simulink model "pattern_separation"  (R2019b)
settings: Solver=FixedStepAuto  StartTime=1  StopTime=simulationtime  FixedStep=stepsize  RelTol=1e-3
values from neighbouring files (symbols this model uses):
  a1 = 0.02    [simulation.m]
  a2 = 0.02    [simulation.m]
  b1 = 0.025    [simulation.m]
  b2 = 0.04    [simulation.m]
  c1 = -65    [simulation.m]
  C1 = normrnd(100,10,[1,nrofgranulecells])    [simulation.m]
  c2 = -65    [simulation.m]
  C2 = normrnd(100,10,[1,nrofinterneurons])    [simulation.m]
  d1 = 6    [simulation.m]
  d2 = 2    [simulation.m]
  inputset = inputsets{no_input}    [simulation.m]
  k1 = 0.25    [simulation.m]
  k2 = 0.25    [simulation.m]
  minimum_saturation_limit_1 = -80    [simulation.m]
  minimum_saturation_limit_2 = -100    [simulation.m]
  noumberofevents = 500    [simulation.m]
  Re = 230    [simulation.m]
  simulationtime = 2000    [simulation.m]
  stepsize = 1    [simulation.m]
  ve1 = -5    [simulation.m]
  ve2 = -80    [simulation.m]
  vr1 = -60    [simulation.m]
  vr2 = -65    [simulation.m]
  vt1 = -55    [simulation.m]
  vt2 = -48    [simulation.m]
undefined symbols (not defined in the file or in its folder): conductancemaxima1, conductancemaxima2, conductancemaxima3, decaytimes1, decaytimes2, decaytimes3, DiscIntNeverNeededParam, Nd, trace
(part 4 of 5)

== system pattern_separation/granule cell 20/GC neuron ==
  postsynaptic current : Inport
  AHP or ADP : Constant  Value=c1  SampleTime=-1
  AP threshold potential : Constant  Value=vt1  SampleTime=-1
  Add : Sum  Inputs=+-
  Add2 : Sum  Inputs=+-
  Add3 : Sum  Inputs=+-
  Constant1 : Constant  Value=d1  SampleTime=-1
  Gain1 : Gain  Gain=b1
  Gain2 : Gain  Gain=k1
  Integrator : Integrator  ExternalReset=rising  InitialCondition=d1
  Integrator1 : Integrator  ExternalReset=rising  InitialCondition=vr1  LimitOutput=on  UpperSaturationLimit=30  LowerSaturationLimit=minimum_saturation_limit_1
  Memory : Memory  InheritSampleTime=on
  Memory1 : Memory  InitialCondition=vr1  InheritSampleTime=on
  Product : Product
  f' : Sum  Inputs=++-
  f'' : Sum  Inputs=+-
  membrne capacitance : Gain  Gain=1/C1(20)
  reset function : MATLAB Function  TreatAsAtomicUnit=on
  resting membrane potential : Constant  Value=vr1  SampleTime=-1
  time constant of relative refractory period : Gain  Gain=a1
  v : Outport
  output : Outport  Port=2
  wires:
  time constant of relative refractory period/1 -> Integrator/1  "u"
  Constant1/1 -> reset function/3(d)
  f''/1 -> time constant of relative refractory period/1
  membrne capacitance/1 -> Integrator1/1  "v"
  resting membrane potential/1 -> Add2/2, Add/2
  AHP or ADP/1 -> reset function/2(c)
  Add2/1 -> Product/1
  reset function/3(r) -> Integrator1/2, Integrator/2, output/1
  Gain1/1 -> f''/1
  Add3/1 -> Product/2
  Memory1/1 -> reset function/1(v)
  reset function/1(v1) -> Add/1, Add2/1, Add3/1
  reset function/2(u1) -> f''/2, f'/3
  Memory/1 -> reset function/4(u)
  Add/1 -> Gain1/1
  Integrator/1 -> Memory/1  "u"
  AP threshold potential/1 -> Add3/2
  Integrator1/1 -> v/1, Memory1/1  "v"
  f'/1 -> membrne capacitance/1
  Product/1 -> Gain2/1
  Gain2/1 -> f'/2
  postsynaptic current/1 -> f'/1

== system pattern_separation/granule cell 20/single exp EPSCs generator (recurrent synapse) ==
  event time : Inport
  decay time constant : Inport  Port=2
  conductance maximum : Inport  Port=3
  Add1 : Sum  Inputs=+-
  MATLAB Function : MATLAB Function  TreatAsAtomicUnit=on
  Multiply : Gain  Gain=-1
  Product : Product
  Product1 : Product  Inputs=*/
  Product2 : Product
  current reversal potential : Constant  Value=ve1  SampleTime=-1
  resting membrane potential : Constant  Value=vr1  SampleTime=-1
  postsynaptic current : Outport
  wires:
  decay time constant/1 -> Product1/2
  Product/1 -> postsynaptic current/1  "postsynaptic current"
  resting membrane potential/1 -> Add1/1
  current reversal potential/1 -> Add1/2
  conductance maximum/1 -> Product2/2
  Product2/1 -> Product/2  "conductance"
  Add1/1 -> Multiply/1
  Product1/1 -> MATLAB Function/1(inp)
  MATLAB Function/1(exponential) -> Product2/1
  event time/1 -> Product1/1
  Multiply/1 -> Product/1

== system pattern_separation/granule cell 20/single exp IPSCs generator (ihibitory synapse) ==
  event time : Inport
  decay time constant : Inport  Port=2
  conductance maximum : Inport  Port=3
  Add1 : Sum  Inputs=+-
  MATLAB Function : MATLAB Function  TreatAsAtomicUnit=on
  Multiply : Gain  Gain=-1
  Product : Product
  Product1 : Product  Inputs=*/
  Product2 : Product
  current reversal potential : Constant  Value=ve2  SampleTime=-1
  resting membrane potential : Constant  Value=vr2  SampleTime=-1
  postsynaptic current : Outport
  wires:
  decay time constant/1 -> Product1/2
  Product/1 -> postsynaptic current/1  "postsynaptic current"
  resting membrane potential/1 -> Add1/1
  current reversal potential/1 -> Add1/2
  conductance maximum/1 -> Product2/2
  Product2/1 -> Product/2  "conductance"
  Add1/1 -> Multiply/1
  Product1/1 -> MATLAB Function/1(inp)
  MATLAB Function/1(exponential) -> Product2/1
  event time/1 -> Product1/1
  Multiply/1 -> Product/1

== system pattern_separation/granule cell 3/GC neuron ==
  postsynaptic current : Inport
  AHP or ADP : Constant  Value=c1  SampleTime=-1
  AP threshold potential : Constant  Value=vt1  SampleTime=-1
  Add : Sum  Inputs=+-
  Add2 : Sum  Inputs=+-
  Add3 : Sum  Inputs=+-
  Constant1 : Constant  Value=d1  SampleTime=-1
  Gain1 : Gain  Gain=b1
  Gain2 : Gain  Gain=k1
  Integrator : Integrator  ExternalReset=rising  InitialCondition=d1
  Integrator1 : Integrator  ExternalReset=rising  InitialCondition=vr1  LimitOutput=on  UpperSaturationLimit=30  LowerSaturationLimit=minimum_saturation_limit_1
  Memory : Memory  InheritSampleTime=on
  Memory1 : Memory  InitialCondition=vr1  InheritSampleTime=on
  Product : Product
  f' : Sum  Inputs=++-
  f'' : Sum  Inputs=+-
  membrne capacitance : Gain  Gain=1/C1(3)
  reset function : MATLAB Function  TreatAsAtomicUnit=on
  resting membrane potential : Constant  Value=vr1  SampleTime=-1
  time constant of relative refractory period : Gain  Gain=a1
  v : Outport
  output : Outport  Port=2
  wires:
  time constant of relative refractory period/1 -> Integrator/1  "u"
  Constant1/1 -> reset function/3(d)
  f''/1 -> time constant of relative refractory period/1
  membrne capacitance/1 -> Integrator1/1  "v"
  resting membrane potential/1 -> Add2/2, Add/2
  AHP or ADP/1 -> reset function/2(c)
  Add2/1 -> Product/1
  reset function/3(r) -> Integrator1/2, Integrator/2, output/1
  Gain1/1 -> f''/1
  Add3/1 -> Product/2
  Memory1/1 -> reset function/1(v)
  reset function/1(v1) -> Add/1, Add2/1, Add3/1
  reset function/2(u1) -> f''/2, f'/3
  Memory/1 -> reset function/4(u)
  Add/1 -> Gain1/1
  Integrator/1 -> Memory/1  "u"
  AP threshold potential/1 -> Add3/2
  Integrator1/1 -> v/1, Memory1/1  "v"
  f'/1 -> membrne capacitance/1
  Product/1 -> Gain2/1
  Gain2/1 -> f'/2
  postsynaptic current/1 -> f'/1

== system pattern_separation/granule cell 3/single exp EPSCs generator (recurrent synapse) ==
  event time : Inport
  decay time constant : Inport  Port=2
  conductance maximum : Inport  Port=3
  Add1 : Sum  Inputs=+-
  MATLAB Function : MATLAB Function  TreatAsAtomicUnit=on
  Multiply : Gain  Gain=-1
  Product : Product
  Product1 : Product  Inputs=*/
  Product2 : Product
  current reversal potential : Constant  Value=ve1  SampleTime=-1
  resting membrane potential : Constant  Value=vr1  SampleTime=-1
  postsynaptic current : Outport
  wires:
  decay time constant/1 -> Product1/2
  Product/1 -> postsynaptic current/1  "postsynaptic current"
  resting membrane potential/1 -> Add1/1
  current reversal potential/1 -> Add1/2
  conductance maximum/1 -> Product2/2
  Product2/1 -> Product/2  "conductance"
  Add1/1 -> Multiply/1
  Product1/1 -> MATLAB Function/1(inp)
  MATLAB Function/1(exponential) -> Product2/1
  event time/1 -> Product1/1
  Multiply/1 -> Product/1

== system pattern_separation/granule cell 3/single exp IPSCs generator (ihibitory synapse) ==
  event time : Inport
  decay time constant : Inport  Port=2
  conductance maximum : Inport  Port=3
  Add1 : Sum  Inputs=+-
  MATLAB Function : MATLAB Function  TreatAsAtomicUnit=on
  Multiply : Gain  Gain=-1
  Product : Product
  Product1 : Product  Inputs=*/
  Product2 : Product
  current reversal potential : Constant  Value=ve2  SampleTime=-1
  resting membrane potential : Constant  Value=vr2  SampleTime=-1
  postsynaptic current : Outport
  wires:
  decay time constant/1 -> Product1/2
  Product/1 -> postsynaptic current/1  "postsynaptic current"
  resting membrane potential/1 -> Add1/1
  current reversal potential/1 -> Add1/2
  conductance maximum/1 -> Product2/2
  Product2/1 -> Product/2  "conductance"
  Add1/1 -> Multiply/1
  Product1/1 -> MATLAB Function/1(inp)
  MATLAB Function/1(exponential) -> Product2/1
  event time/1 -> Product1/1
  Multiply/1 -> Product/1

== system pattern_separation/granule cell 4/GC neuron ==
  postsynaptic current : Inport
  AHP or ADP : Constant  Value=c1  SampleTime=-1
  AP threshold potential : Constant  Value=vt1  SampleTime=-1
  Add : Sum  Inputs=+-
  Add2 : Sum  Inputs=+-
  Add3 : Sum  Inputs=+-
  Constant1 : Constant  Value=d1  SampleTime=-1
  Gain1 : Gain  Gain=b1
  Gain2 : Gain  Gain=k1
  Integrator : Integrator  ExternalReset=rising  InitialCondition=d1
  Integrator1 : Integrator  ExternalReset=rising  InitialCondition=vr1  LimitOutput=on  UpperSaturationLimit=30  LowerSaturationLimit=minimum_saturation_limit_1
  Memory : Memory  InheritSampleTime=on
  Memory1 : Memory  InitialCondition=vr1  InheritSampleTime=on
  Product : Product
  f' : Sum  Inputs=++-
  f'' : Sum  Inputs=+-
  membrne capacitance : Gain  Gain=1/C1(4)
  reset function : MATLAB Function  TreatAsAtomicUnit=on
  resting membrane potential : Constant  Value=vr1  SampleTime=-1
  time constant of relative refractory period : Gain  Gain=a1
  v : Outport
  output : Outport  Port=2
  wires:
  time constant of relative refractory period/1 -> Integrator/1  "u"
  Constant1/1 -> reset function/3(d)
  f''/1 -> time constant of relative refractory period/1
  membrne capacitance/1 -> Integrator1/1  "v"
  resting membrane potential/1 -> Add2/2, Add/2
  AHP or ADP/1 -> reset function/2(c)
  Add2/1 -> Product/1
  reset function/3(r) -> Integrator1/2, Integrator/2, output/1
  Gain1/1 -> f''/1
  Add3/1 -> Product/2
  Memory1/1 -> reset function/1(v)
  reset function/1(v1) -> Add/1, Add2/1, Add3/1
  reset function/2(u1) -> f''/2, f'/3
  Memory/1 -> reset function/4(u)
  Add/1 -> Gain1/1
  Integrator/1 -> Memory/1  "u"
  AP threshold potential/1 -> Add3/2
  Integrator1/1 -> v/1, Memory1/1  "v"
  f'/1 -> membrne capacitance/1
  Product/1 -> Gain2/1
  Gain2/1 -> f'/2
  postsynaptic current/1 -> f'/1

== system pattern_separation/granule cell 4/single exp EPSCs generator (recurrent synapse) ==
  event time : Inport
  decay time constant : Inport  Port=2
  conductance maximum : Inport  Port=3
  Add1 : Sum  Inputs=+-
  MATLAB Function : MATLAB Function  TreatAsAtomicUnit=on
  Multiply : Gain  Gain=-1
  Product : Product
  Product1 : Product  Inputs=*/
  Product2 : Product
  current reversal potential : Constant  Value=ve1  SampleTime=-1
  resting membrane potential : Constant  Value=vr1  SampleTime=-1
  postsynaptic current : Outport
  wires:
  decay time constant/1 -> Product1/2
  Product/1 -> postsynaptic current/1  "postsynaptic current"
  resting membrane potential/1 -> Add1/1
  current reversal potential/1 -> Add1/2
  conductance maximum/1 -> Product2/2
  Product2/1 -> Product/2  "conductance"
  Add1/1 -> Multiply/1
  Product1/1 -> MATLAB Function/1(inp)
  MATLAB Function/1(exponential) -> Product2/1
  event time/1 -> Product1/1
  Multiply/1 -> Product/1

== system pattern_separation/granule cell 4/single exp IPSCs generator (ihibitory synapse) ==
  event time : Inport
  decay time constant : Inport  Port=2
  conductance maximum : Inport  Port=3
  Add1 : Sum  Inputs=+-
  MATLAB Function : MATLAB Function  TreatAsAtomicUnit=on
  Multiply : Gain  Gain=-1
  Product : Product
  Product1 : Product  Inputs=*/
  Product2 : Product
  current reversal potential : Constant  Value=ve2  SampleTime=-1
  resting membrane potential : Constant  Value=vr2  SampleTime=-1
  postsynaptic current : Outport
  wires:
  decay time constant/1 -> Product1/2
  Product/1 -> postsynaptic current/1  "postsynaptic current"
  resting membrane potential/1 -> Add1/1
  current reversal potential/1 -> Add1/2
  conductance maximum/1 -> Product2/2
  Product2/1 -> Product/2  "conductance"
  Add1/1 -> Multiply/1
  Product1/1 -> MATLAB Function/1(inp)
  MATLAB Function/1(exponential) -> Product2/1
  event time/1 -> Product1/1
  Multiply/1 -> Product/1

== system pattern_separation/granule cell 5/granule cell ==
  postsynaptic current : Inport
  AHP or ADP : Constant  Value=c1  SampleTime=-1
  AP threshold potential : Constant  Value=vt1  SampleTime=-1
  Add : Sum  Inputs=+-
  Add2 : Sum  Inputs=+-
  Add3 : Sum  Inputs=+-
  Constant1 : Constant  Value=d1  SampleTime=-1
  Gain1 : Gain  Gain=b1
  Gain2 : Gain  Gain=k1
  Integrator : Integrator  ExternalReset=rising  InitialCondition=d1
  Integrator1 : Integrator  ExternalReset=rising  InitialCondition=vr1  LimitOutput=on  UpperSaturationLimit=30  LowerSaturationLimit=minimum_saturation_limit_1
  Memory : Memory  InheritSampleTime=on
  Memory1 : Memory  InitialCondition=vr1  InheritSampleTime=on
  Product : Product
  f' : Sum  Inputs=++-
  f'' : Sum  Inputs=+-
  membrne capacitance : Gain  Gain=1/C1(5)
  reset function : MATLAB Function  TreatAsAtomicUnit=on
  resting membrane potential : Constant  Value=vr1  SampleTime=-1
  time constant of relative refractory period : Gain  Gain=a1
  v : Outport
  output : Outport  Port=2
  wires:
  time constant of relative refractory period/1 -> Integrator/1  "u"
  Constant1/1 -> reset function/3(d)
  f''/1 -> time constant of relative refractory period/1
  membrne capacitance/1 -> Integrator1/1  "v"
  resting membrane potential/1 -> Add2/2, Add/2
  AHP or ADP/1 -> reset function/2(c)
  Add2/1 -> Product/1
  reset function/3(r) -> output/1, Integrator1/2, Integrator/2
  Gain1/1 -> f''/1
  Add3/1 -> Product/2
  Memory1/1 -> reset function/1(v)
  reset function/1(v1) -> Add/1, Add2/1, Add3/1
  reset function/2(u1) -> f''/2, f'/3
  Memory/1 -> reset function/4(u)
  Add/1 -> Gain1/1
  Integrator/1 -> Memory/1  "u"
  AP threshold potential/1 -> Add3/2
  Integrator1/1 -> v/1, Memory1/1  "v"
  f'/1 -> membrne capacitance/1
  Product/1 -> Gain2/1
  Gain2/1 -> f'/2
  postsynaptic current/1 -> f'/1

== system pattern_separation/granule cell 5/single exp EPSCs generator (recurrent synapse) ==
  event time : Inport
  decay time constant : Inport  Port=2
  conductance maximum : Inport  Port=3
  Add1 : Sum  Inputs=+-
  MATLAB Function : MATLAB Function  TreatAsAtomicUnit=on
  Multiply : Gain  Gain=-1
  Product : Product
  Product1 : Product  Inputs=*/
  Product2 : Product
  current reversal potential : Constant  Value=ve1  SampleTime=-1
  resting membrane potential : Constant  Value=vr1  SampleTime=-1
  postsynaptic current : Outport
  wires:
  decay time constant/1 -> Product1/2
  Product/1 -> postsynaptic current/1  "postsynaptic current"
  resting membrane potential/1 -> Add1/1
  current reversal potential/1 -> Add1/2
  conductance maximum/1 -> Product2/2
  Product2/1 -> Product/2  "conductance"
  Add1/1 -> Multiply/1
  Product1/1 -> MATLAB Function/1(inp)
  MATLAB Function/1(exponential) -> Product2/1
  event time/1 -> Product1/1
  Multiply/1 -> Product/1

== system pattern_separation/granule cell 5/single exp IPSCs generator (ihibitory synapse) ==
  event time : Inport
  decay time constant : Inport  Port=2
  conductance maximum : Inport  Port=3
  Add1 : Sum  Inputs=+-
  MATLAB Function : MATLAB Function  TreatAsAtomicUnit=on
  Multiply : Gain  Gain=-1
  Product : Product
  Product1 : Product  Inputs=*/
  Product2 : Product
  current reversal potential : Constant  Value=ve2  SampleTime=-1
  resting membrane potential : Constant  Value=vr2  SampleTime=-1
  postsynaptic current : Outport
  wires:
  decay time constant/1 -> Product1/2
  Product/1 -> postsynaptic current/1  "postsynaptic current"
  resting membrane potential/1 -> Add1/1
  current reversal potential/1 -> Add1/2
  conductance maximum/1 -> Product2/2
  Product2/1 -> Product/2  "conductance"
  Add1/1 -> Multiply/1
  Product1/1 -> MATLAB Function/1(inp)
  MATLAB Function/1(exponential) -> Product2/1
  event time/1 -> Product1/1
  Multiply/1 -> Product/1

== system pattern_separation/granule cell 6/GC neuron ==
  postsynaptic current : Inport
  AHP or ADP : Constant  Value=c1  SampleTime=-1
  AP threshold potential : Constant  Value=vt1  SampleTime=-1
  Add : Sum  Inputs=+-
  Add2 : Sum  Inputs=+-
  Add3 : Sum  Inputs=+-
  Constant1 : Constant  Value=d1  SampleTime=-1
  Gain1 : Gain  Gain=b1
  Gain2 : Gain  Gain=k1
  Integrator : Integrator  ExternalReset=rising  InitialCondition=d1
  Integrator1 : Integrator  ExternalReset=rising  InitialCondition=vr1  LimitOutput=on  UpperSaturationLimit=30  LowerSaturationLimit=minimum_saturation_limit_1
  Memory : Memory  InheritSampleTime=on
  Memory1 : Memory  InitialCondition=vr1  InheritSampleTime=on
  Product : Product  RndMeth=Nearest
  f' : Sum  Inputs=++-
  f'' : Sum  Inputs=+-
  membrne capacitance : Gain  Gain=1/C1(6)
  reset function : MATLAB Function  TreatAsAtomicUnit=on
  resting membrane potential : Constant  Value=vr1  SampleTime=-1
  time constant of relative refractory period : Gain  Gain=a1
  v : Outport
  output : Outport  Port=2
  wires:
  time constant of relative refractory period/1 -> Integrator/1  "u"
  Constant1/1 -> reset function/3(d)
  f''/1 -> time constant of relative refractory period/1
  membrne capacitance/1 -> Integrator1/1  "v"
  resting membrane potential/1 -> Add2/2, Add/2
  AHP or ADP/1 -> reset function/2(c)
  Add2/1 -> Product/1
  reset function/3(r) -> Integrator1/2, Integrator/2, output/1
  Gain1/1 -> f''/1
  Add3/1 -> Product/2
  Memory1/1 -> reset function/1(v)
  reset function/1(v1) -> Add/1, Add2/1, Add3/1
  reset function/2(u1) -> f''/2, f'/3
  Memory/1 -> reset function/4(u)
  Add/1 -> Gain1/1
  Integrator/1 -> Memory/1  "u"
  AP threshold potential/1 -> Add3/2
  Integrator1/1 -> v/1, Memory1/1  "v"
  f'/1 -> membrne capacitance/1
  Product/1 -> Gain2/1
  Gain2/1 -> f'/2
  postsynaptic current/1 -> f'/1

== system pattern_separation/granule cell 6/single exp EPSCs generator (recurrent synapse) ==
  event time : Inport
  decay time constant : Inport  Port=2
  conductance maximum : Inport  Port=3
  Add1 : Sum  Inputs=+-
  MATLAB Function : MATLAB Function  TreatAsAtomicUnit=on
  Multiply : Gain  Gain=-1
  Product : Product
  Product1 : Product  Inputs=*/
  Product2 : Product
  current reversal potential : Constant  Value=ve1  SampleTime=-1
  resting membrane potential : Constant  Value=vr1  SampleTime=-1
  postsynaptic current : Outport
  wires:
  decay time constant/1 -> Product1/2
  Product/1 -> postsynaptic current/1  "postsynaptic current"
  resting membrane potential/1 -> Add1/1
  current reversal potential/1 -> Add1/2
  conductance maximum/1 -> Product2/2
  Product2/1 -> Product/2  "conductance"
  Add1/1 -> Multiply/1
  Product1/1 -> MATLAB Function/1(inp)
  MATLAB Function/1(exponential) -> Product2/1
  event time/1 -> Product1/1
  Multiply/1 -> Product/1

== system pattern_separation/granule cell 6/single exp IPSCs generator (ihibitory synapse) ==
  event time : Inport
  decay time constant : Inport  Port=2
  conductance maximum : Inport  Port=3
  Add1 : Sum  Inputs=+-
  MATLAB Function : MATLAB Function  TreatAsAtomicUnit=on
  Multiply : Gain  Gain=-1
  Product : Product
  Product1 : Product  Inputs=*/
  Product2 : Product
  current reversal potential : Constant  Value=ve2  SampleTime=-1
  resting membrane potential : Constant  Value=vr2  SampleTime=-1
  postsynaptic current : Outport
  wires:
  decay time constant/1 -> Product1/2
  Product/1 -> postsynaptic current/1  "postsynaptic current"
  resting membrane potential/1 -> Add1/1
  current reversal potential/1 -> Add1/2
  conductance maximum/1 -> Product2/2
  Product2/1 -> Product/2  "conductance"
  Add1/1 -> Multiply/1
  Product1/1 -> MATLAB Function/1(inp)
  MATLAB Function/1(exponential) -> Product2/1
  event time/1 -> Product1/1
  Multiply/1 -> Product/1

== system pattern_separation/granule cell 7/granule cell ==
  postsynaptic current : Inport
  AHP or ADP : Constant  Value=c1  SampleTime=-1
  AP threshold potential : Constant  Value=vt1  SampleTime=-1
  Add : Sum  Inputs=+-
  Add2 : Sum  Inputs=+-
  Add3 : Sum  Inputs=+-
  Constant1 : Constant  Value=d1  SampleTime=-1
  Gain1 : Gain  Gain=b1
  Gain2 : Gain  Gain=k1
  Integrator : Integrator  ExternalReset=rising  InitialCondition=d1
  Integrator1 : Integrator  ExternalReset=rising  InitialCondition=vr1  LimitOutput=on  UpperSaturationLimit=30  LowerSaturationLimit=minimum_saturation_limit_1
  Memory : Memory  InheritSampleTime=on
  Memory1 : Memory  InitialCondition=vr1  InheritSampleTime=on
  Product : Product
  f' : Sum  Inputs=++-
  f'' : Sum  Inputs=+-
  membrne capacitance : Gain  Gain=1/C1(7)
  reset function : MATLAB Function  TreatAsAtomicUnit=on
  resting membrane potential : Constant  Value=vr1  SampleTime=-1
  time constant of relative refractory period : Gain  Gain=a1
  v : Outport
  output : Outport  Port=2
  wires:
  time constant of relative refractory period/1 -> Integrator/1  "u"
  Constant1/1 -> reset function/3(d)
  f''/1 -> time constant of relative refractory period/1
  membrne capacitance/1 -> Integrator1/1  "v"
  resting membrane potential/1 -> Add2/2, Add/2
  AHP or ADP/1 -> reset function/2(c)
  Add2/1 -> Product/1
  reset function/3(r) -> output/1, Integrator1/2, Integrator/2
  Gain1/1 -> f''/1
  Add3/1 -> Product/2
  Memory1/1 -> reset function/1(v)
  reset function/1(v1) -> Add/1, Add2/1, Add3/1
  reset function/2(u1) -> f''/2, f'/3
  Memory/1 -> reset function/4(u)
  Add/1 -> Gain1/1
  Integrator/1 -> Memory/1  "u"
  AP threshold potential/1 -> Add3/2
  Integrator1/1 -> v/1, Memory1/1  "v"
  f'/1 -> membrne capacitance/1
  Product/1 -> Gain2/1
  Gain2/1 -> f'/2
  postsynaptic current/1 -> f'/1

== system pattern_separation/granule cell 7/single exp EPSCs generator (recurrent synapse) ==
  event time : Inport
  decay time constant : Inport  Port=2
  conductance maximum : Inport  Port=3
  Add1 : Sum  Inputs=+-
  MATLAB Function : MATLAB Function  TreatAsAtomicUnit=on
  Multiply : Gain  Gain=-1
  Product : Product
  Product1 : Product  Inputs=*/
  Product2 : Product
  current reversal potential : Constant  Value=ve1  SampleTime=-1
  resting membrane potential : Constant  Value=vr1  SampleTime=-1
  postsynaptic current : Outport
  wires:
  decay time constant/1 -> Product1/2
  Product/1 -> postsynaptic current/1  "postsynaptic current"
  resting membrane potential/1 -> Add1/1
  current reversal potential/1 -> Add1/2
  conductance maximum/1 -> Product2/2
  Product2/1 -> Product/2  "conductance"
  Add1/1 -> Multiply/1
  Product1/1 -> MATLAB Function/1(inp)
  MATLAB Function/1(exponential) -> Product2/1
  event time/1 -> Product1/1
  Multiply/1 -> Product/1

== system pattern_separation/granule cell 7/single exp IPSCs generator (ihibitory synapse) ==
  event time : Inport
  decay time constant : Inport  Port=2
  conductance maximum : Inport  Port=3
  Add1 : Sum  Inputs=+-
  MATLAB Function : MATLAB Function  TreatAsAtomicUnit=on
  Multiply : Gain  Gain=-1
  Product : Product
  Product1 : Product  Inputs=*/
  Product2 : Product
  current reversal potential : Constant  Value=ve2  SampleTime=-1
  resting membrane potential : Constant  Value=vr2  SampleTime=-1
  postsynaptic current : Outport
  wires:
  decay time constant/1 -> Product1/2
  Product/1 -> postsynaptic current/1  "postsynaptic current"
  resting membrane potential/1 -> Add1/1
  current reversal potential/1 -> Add1/2
  conductance maximum/1 -> Product2/2
  Product2/1 -> Product/2  "conductance"
  Add1/1 -> Multiply/1
  Product1/1 -> MATLAB Function/1(inp)
  MATLAB Function/1(exponential) -> Product2/1
  event time/1 -> Product1/1
  Multiply/1 -> Product/1

== system pattern_separation/granule cell 8/GC neuron ==
  postsynaptic current : Inport
  AHP or ADP : Constant  Value=c1  SampleTime=-1
  AP threshold potential : Constant  Value=vt1  SampleTime=-1
  Add : Sum  Inputs=+-
  Add2 : Sum  Inputs=+-
  Add3 : Sum  Inputs=+-
  Constant1 : Constant  Value=d1  SampleTime=-1
  Gain1 : Gain  Gain=b1
  Gain2 : Gain  Gain=k1
  Integrator : Integrator  ExternalReset=rising  InitialCondition=d1
  Integrator1 : Integrator  ExternalReset=rising  InitialCondition=vr1  LimitOutput=on  UpperSaturationLimit=30  LowerSaturationLimit=minimum_saturation_limit_1
  Memory : Memory  InheritSampleTime=on
  Memory1 : Memory  InitialCondition=vr1  InheritSampleTime=on
  Product : Product
  f' : Sum  Inputs=++-
  f'' : Sum  Inputs=+-
  membrne capacitance : Gain  Gain=1/C1(8)
  reset function : MATLAB Function  TreatAsAtomicUnit=on
  resting membrane potential : Constant  Value=vr1  SampleTime=-1
  time constant of relative refractory period : Gain  Gain=a1
  v : Outport
  output : Outport  Port=2
  wires:
  time constant of relative refractory period/1 -> Integrator/1  "u"
  Constant1/1 -> reset function/3(d)
  f''/1 -> time constant of relative refractory period/1
  membrne capacitance/1 -> Integrator1/1  "v"
  resting membrane potential/1 -> Add2/2, Add/2
  AHP or ADP/1 -> reset function/2(c)
  Add2/1 -> Product/1
  reset function/3(r) -> Integrator1/2, Integrator/2, output/1
  Gain1/1 -> f''/1
  Add3/1 -> Product/2
  Memory1/1 -> reset function/1(v)
  reset function/1(v1) -> Add/1, Add2/1, Add3/1
  reset function/2(u1) -> f''/2, f'/3
  Memory/1 -> reset function/4(u)
  Add/1 -> Gain1/1
  Integrator/1 -> Memory/1  "u"
  AP threshold potential/1 -> Add3/2
  Integrator1/1 -> v/1, Memory1/1  "v"
  f'/1 -> membrne capacitance/1
  Product/1 -> Gain2/1
  Gain2/1 -> f'/2
  postsynaptic current/1 -> f'/1

== system pattern_separation/granule cell 8/single exp EPSCs generator (recurrent synapse) ==
  event time : Inport
  decay time constant : Inport  Port=2
  conductance maximum : Inport  Port=3
  Add1 : Sum  Inputs=+-
  MATLAB Function : MATLAB Function  TreatAsAtomicUnit=on
  Multiply : Gain  Gain=-1
  Product : Product
  Product1 : Product  Inputs=*/
  Product2 : Product
  current reversal potential : Constant  Value=ve1  SampleTime=-1
  resting membrane potential : Constant  Value=vr1  SampleTime=-1
  postsynaptic current : Outport
  wires:
  decay time constant/1 -> Product1/2
  Product/1 -> postsynaptic current/1  "postsynaptic current"
  resting membrane potential/1 -> Add1/1
  current reversal potential/1 -> Add1/2
  conductance maximum/1 -> Product2/2
  Product2/1 -> Product/2  "conductance"
  Add1/1 -> Multiply/1
  Product1/1 -> MATLAB Function/1(inp)
  MATLAB Function/1(exponential) -> Product2/1
  event time/1 -> Product1/1
  Multiply/1 -> Product/1

== system pattern_separation/granule cell 8/single exp IPSCs generator (ihibitory synapse) ==
  event time : Inport
  decay time constant : Inport  Port=2
  conductance maximum : Inport  Port=3
  Add1 : Sum  Inputs=+-
  MATLAB Function : MATLAB Function  TreatAsAtomicUnit=on
  Multiply : Gain  Gain=-1
  Product : Product
  Product1 : Product  Inputs=*/
  Product2 : Product
  current reversal potential : Constant  Value=ve2  SampleTime=-1
  resting membrane potential : Constant  Value=vr2  SampleTime=-1
  postsynaptic current : Outport
  wires:
  decay time constant/1 -> Product1/2
  Product/1 -> postsynaptic current/1  "postsynaptic current"
  resting membrane potential/1 -> Add1/1
  current reversal potential/1 -> Add1/2
  conductance maximum/1 -> Product2/2
  Product2/1 -> Product/2  "conductance"
  Add1/1 -> Multiply/1
  Product1/1 -> MATLAB Function/1(inp)
  MATLAB Function/1(exponential) -> Product2/1
  event time/1 -> Product1/1
  Multiply/1 -> Product/1

== system pattern_separation/granule cell 9/granule cell ==
  postsynaptic current : Inport
  AHP or ADP : Constant  Value=c1  SampleTime=-1
  AP threshold potential : Constant  Value=vt1  SampleTime=-1
  Add : Sum  Inputs=+-
  Add2 : Sum  Inputs=+-
  Add3 : Sum  Inputs=+-
  Constant1 : Constant  Value=d1  SampleTime=-1
  Gain1 : Gain  Gain=b1
  Gain2 : Gain  Gain=k1
  Integrator : Integrator  ExternalReset=rising  InitialCondition=d1
  Integrator1 : Integrator  ExternalReset=rising  InitialCondition=vr1  LimitOutput=on  UpperSaturationLimit=30  LowerSaturationLimit=minimum_saturation_limit_1
  Memory : Memory  InheritSampleTime=on
  Memory1 : Memory  InitialCondition=vr1  InheritSampleTime=on
  Product : Product
  f' : Sum  Inputs=++-
  f'' : Sum  Inputs=+-
  membrne capacitance : Gain  Gain=1/C1(9)
  reset function : MATLAB Function  TreatAsAtomicUnit=on
  resting membrane potential : Constant  Value=vr1  SampleTime=-1
  time constant of relative refractory period : Gain  Gain=a1
  v : Outport
  output : Outport  Port=2
  wires:
  time constant of relative refractory period/1 -> Integrator/1  "u"
  Constant1/1 -> reset function/3(d)
  f''/1 -> time constant of relative refractory period/1
  membrne capacitance/1 -> Integrator1/1  "v"
  resting membrane potential/1 -> Add2/2, Add/2
  AHP or ADP/1 -> reset function/2(c)
  Add2/1 -> Product/1
  reset function/3(r) -> output/1, Integrator1/2, Integrator/2
  Gain1/1 -> f''/1
  Add3/1 -> Product/2
  Memory1/1 -> reset function/1(v)
  reset function/1(v1) -> Add/1, Add2/1, Add3/1
  reset function/2(u1) -> f''/2, f'/3
  Memory/1 -> reset function/4(u)
  Add/1 -> Gain1/1
  Integrator/1 -> Memory/1  "u"
  AP threshold potential/1 -> Add3/2
  Integrator1/1 -> v/1, Memory1/1  "v"
  f'/1 -> membrne capacitance/1
  Product/1 -> Gain2/1
  Gain2/1 -> f'/2
  postsynaptic current/1 -> f'/1

== system pattern_separation/granule cell 9/single exp EPSCs generator (recurrent synapse) ==
  event time : Inport
  decay time constant : Inport  Port=2
  conductance maximum : Inport  Port=3
  Add1 : Sum  Inputs=+-
  MATLAB Function : MATLAB Function  TreatAsAtomicUnit=on
  Multiply : Gain  Gain=-1
  Product : Product
  Product1 : Product  Inputs=*/
  Product2 : Product
  current reversal potential : Constant  Value=ve1  SampleTime=-1
  resting membrane potential : Constant  Value=vr1  SampleTime=-1
  postsynaptic current : Outport
  wires:
  decay time constant/1 -> Product1/2
  Product/1 -> postsynaptic current/1  "postsynaptic current"
  resting membrane potential/1 -> Add1/1
  current reversal potential/1 -> Add1/2
  conductance maximum/1 -> Product2/2
  Product2/1 -> Product/2  "conductance"
  Add1/1 -> Multiply/1
  Product1/1 -> MATLAB Function/1(inp)
  MATLAB Function/1(exponential) -> Product2/1
  event time/1 -> Product1/1
  Multiply/1 -> Product/1

== system pattern_separation/granule cell 9/single exp IPSCs generator (ihibitory synapse) ==
  event time : Inport
  decay time constant : Inport  Port=2
  conductance maximum : Inport  Port=3
  Add1 : Sum  Inputs=+-
  MATLAB Function : MATLAB Function  TreatAsAtomicUnit=on
  Multiply : Gain  Gain=-1
  Product : Product
  Product1 : Product  Inputs=*/
  Product2 : Product
  current reversal potential : Constant  Value=ve2  SampleTime=-1
  resting membrane potential : Constant  Value=vr2  SampleTime=-1
  postsynaptic current : Outport
  wires:
  decay time constant/1 -> Product1/2
  Product/1 -> postsynaptic current/1  "postsynaptic current"
  resting membrane potential/1 -> Add1/1
  current reversal potential/1 -> Add1/2
  conductance maximum/1 -> Product2/2
  Product2/1 -> Product/2  "conductance"
  Add1/1 -> Multiply/1
  Product1/1 -> MATLAB Function/1(inp)
  MATLAB Function/1(exponential) -> Product2/1
  event time/1 -> Product1/1
  Multiply/1 -> Product/1

== matlab function pattern_separation/granule cell 2/MATLAB Function1 ==
  data: eventnoumber input; decaytime output; decaytimes1 input; conductancemaxima1 input; conductancemaximum output
function [decaytime, conductancemaximum] = fcn(eventnoumber, decaytimes1, conductancemaxima1)
if eventnoumber ==0
decaytime =1;
conductancemaximum =0;
else
decaytime = decaytimes1(2, eventnoumber);
conductancemaximum = conductancemaxima1(2, eventnoumber);
end

== matlab function pattern_separation/granule cell 2/MATLAB Function2 ==
  data: eventnoumber input; decaytime output; decaytimes2 input; conductancemaxima2 input; conductancemaximum output
function [decaytime, conductancemaximum] = fcn(eventnoumber, decaytimes2, conductancemaxima2)
if eventnoumber ==0
decaytime =1;
conductancemaximum =0;
else
decaytime = decaytimes2(2, eventnoumber);
conductancemaximum = conductancemaxima2(2, eventnoumber);
end

== matlab function pattern_separation/granule cell 2/single exp EPSCs generator (recurrent synapse)/MATLAB Function ==
  data: inp input; exponential output
function exponential = fcn(inp)

exponential = exp(-inp);

== matlab function pattern_separation/granule cell 2/single exp IPSCs generator (ihibitory synapse)/MATLAB Function ==
  data: inp input; exponential output
function exponential = fcn(inp)

exponential = exp(-inp);

== matlab function pattern_separation/granule cell 2/GC neuron/reset function ==
  data: v input; c input; d input; u input; v1 output; u1 output; r output

function [v1,u1,r] = fcn(v,c,d,u)

if v >= 30
v1= c;
u1 = u+d;
r=1;
else
v1=v;
u1=u;
r=0;  
end

== matlab function pattern_separation/granule cell 3/GC neuron/reset function ==
  data: v input; c input; d input; u input; v1 output; u1 output; r output

function [v1,u1,r] = fcn(v,c,d,u)

if v >= 30
v1= c;
u1 = u+d;
r=1;
else
v1=v;
u1=u;
r=0;  
end

== matlab function pattern_separation/PV+ interneuron 1/MATLAB Function1 ==
  data: eventnoumber input; decaytime output; decaytimes3 input; conductancemaxima3 input; conductancemaximum output
function [decaytime, conductancemaximum] = fcn(eventnoumber, decaytimes3, conductancemaxima3)
if eventnoumber ==0
decaytime =1;
conductancemaximum =0;
else
decaytime = decaytimes3(1, eventnoumber);
conductancemaximum = conductancemaxima3(1, eventnoumber);
end

== matlab function pattern_separation/PV+ interneuron 1/interneuron/reset function ==
  data: v input; c input; d input; u input; v1 output; u1 output; r output

function [v1,u1,r] = fcn(v,c,d,u)

if v >= 30
v1= c;
u1 = u+d;
r=1;
else
v1=v;
u1=u;
r=0;  
end

== matlab function pattern_separation/PV+ interneuron 1/single exp EPSCs generator (ff synapse)/MATLAB Function ==
  data: inp input; exponential output
function exponential = fcn(inp)

exponential = exp(-inp);

== matlab function pattern_separation/granule cell 3/MATLAB Function1 ==
  data: eventnoumber input; decaytime output; decaytimes1 input; conductancemaxima1 input; conductancemaximum output
function [decaytime, conductancemaximum] = fcn(eventnoumber, decaytimes1, conductancemaxima1)
if eventnoumber ==0
decaytime =1;
conductancemaximum =0;
else
decaytime = decaytimes1(3, eventnoumber);
conductancemaximum = conductancemaxima1(3, eventnoumber);
end

== matlab function pattern_separation/granule cell 3/MATLAB Function2 ==
  data: eventnoumber input; decaytime output; decaytimes2 input; conductancemaxima2 input; conductancemaximum output
function [decaytime, conductancemaximum] = fcn(eventnoumber, decaytimes2, conductancemaxima2)
if eventnoumber ==0
decaytime =1;
conductancemaximum =0;
else
decaytime = decaytimes2(3, eventnoumber);
conductancemaximum = conductancemaxima2(3, eventnoumber);
end

== matlab function pattern_separation/granule cell 3/single exp EPSCs generator (recurrent synapse)/MATLAB Function ==
  data: inp input; exponential output
function exponential = fcn(inp)

exponential = exp(-inp);

== matlab function pattern_separation/granule cell 3/single exp IPSCs generator (ihibitory synapse)/MATLAB Function ==
  data: inp input; exponential output
function exponential = fcn(inp)

exponential = exp(-inp);

== matlab function pattern_separation/granule cell 1/granule cell/reset function ==
  data: v input; c input; d input; u input; v1 output; u1 output; r output

function [v1,u1,r] = fcn(v,c,d,u)

if v >= 30
v1= c;
u1 = u+d;
r=1;
else
v1=v;
u1=u;
r=0;  
end

== matlab function pattern_separation/granule cell 4/GC neuron/reset function ==
  data: v input; c input; d input; u input; v1 output; u1 output; r output

function [v1,u1,r] = fcn(v,c,d,u)

if v >= 30
v1= c;
u1 = u+d;
r=1;
else
v1=v;
u1=u;
r=0;  
end

== matlab function pattern_separation/granule cell 4/MATLAB Function1 ==
  data: eventnoumber input; decaytime output; decaytimes1 input; conductancemaxima1 input; conductancemaximum output
function [decaytime, conductancemaximum] = fcn(eventnoumber, decaytimes1, conductancemaxima1)
if eventnoumber ==0
decaytime =1;
conductancemaximum =0;
else
decaytime = decaytimes1(4, eventnoumber);
conductancemaximum = conductancemaxima1(4, eventnoumber);
end

== matlab function pattern_separation/granule cell 4/MATLAB Function2 ==
  data: eventnoumber input; decaytime output; decaytimes2 input; conductancemaxima2 input; conductancemaximum output
function [decaytime, conductancemaximum] = fcn(eventnoumber, decaytimes2, conductancemaxima2)
if eventnoumber ==0
decaytime =1;
conductancemaximum =0;
else
decaytime = decaytimes2(4, eventnoumber);
conductancemaximum = conductancemaxima2(4, eventnoumber);
end

== matlab function pattern_separation/granule cell 4/single exp EPSCs generator (recurrent synapse)/MATLAB Function ==
  data: inp input; exponential output
function exponential = fcn(inp)

exponential = exp(-inp);

== matlab function pattern_separation/granule cell 4/single exp IPSCs generator (ihibitory synapse)/MATLAB Function ==
  data: inp input; exponential output
function exponential = fcn(inp)

exponential = exp(-inp);

== matlab function pattern_separation/PV+ interneuron 2/MATLAB Function1 ==
  data: eventnoumber input; decaytime output; decaytimes3 input; conductancemaxima3 input; conductancemaximum output
function [decaytime, conductancemaximum] = fcn(eventnoumber, decaytimes3, conductancemaxima3)
if eventnoumber ==0
decaytime =1;
conductancemaximum =0;
else
decaytime = decaytimes3(2,eventnoumber);
conductancemaximum = conductancemaxima3(2,eventnoumber);
end

== matlab function pattern_separation/PV+ interneuron 2/interneuron/reset function ==
  data: v input; c input; d input; u input; v1 output; u1 output; r output

function [v1,u1,r] = fcn(v,c,d,u)

if v >= 30
v1= c;
u1 = u+d;
r=1;
else
v1=v;
u1=u;
r=0;  
end

== matlab function pattern_separation/PV+ interneuron 2/single exp EPSCs generator (ff synapse)/MATLAB Function ==
  data: inp input; exponential output
function exponential = fcn(inp)

exponential = exp(-inp);

== matlab function pattern_separation/granule cell 5/MATLAB Function1 ==
  data: eventnoumber input; decaytime output; decaytimes1 input; conductancemaxima1 input; conductancemaximum output
function [decaytime, conductancemaximum] = fcn(eventnoumber, decaytimes1, conductancemaxima1)
if eventnoumber ==0
decaytime =1;
conductancemaximum =0;
else
decaytime = decaytimes1(5, eventnoumber);
conductancemaximum = conductancemaxima1(5, eventnoumber);
end

== matlab function pattern_separation/granule cell 5/MATLAB Function2 ==
  data: eventnoumber input; decaytime output; decaytimes2 input; conductancemaxima2 input; conductancemaximum output
function [decaytime, conductancemaximum] = fcn(eventnoumber, decaytimes2, conductancemaxima2)
if eventnoumber ==0
decaytime =1;
conductancemaximum =0;
else
decaytime = decaytimes2(5, eventnoumber);
conductancemaximum = conductancemaxima2(5, eventnoumber);
end

== matlab function pattern_separation/granule cell 5/granule cell/reset function ==
  data: v input; c input; d input; u input; v1 output; u1 output; r output

function [v1,u1,r] = fcn(v,c,d,u)

if v >= 30
v1= c;
u1 = u+d;
r=1;
else
v1=v;
u1=u;
r=0;  
end

== matlab function pattern_separation/granule cell 5/single exp EPSCs generator (recurrent synapse)/MATLAB Function ==
  data: inp input; exponential output
function exponential = fcn(inp)

exponential = exp(-inp);

== matlab function pattern_separation/granule cell 5/single exp IPSCs generator (ihibitory synapse)/MATLAB Function ==
  data: inp input; exponential output
function exponential = fcn(inp)

exponential = exp(-inp);

== matlab function pattern_separation/granule cell 6/GC neuron/reset function ==
  data: v input; c input; d input; u input; v1 output; u1 output; r output

function [v1,u1,r] = fcn(v,c,d,u)

if v >= 30
v1= c;
u1 = u+d;
r=1;
else
v1=v;
u1=u;
r=0;  
end

== matlab function pattern_separation/granule cell 6/MATLAB Function1 ==
  data: eventnoumber input; decaytime output; decaytimes1 input; conductancemaxima1 input; conductancemaximum output
function [decaytime, conductancemaximum] = fcn(eventnoumber, decaytimes1, conductancemaxima1)
if eventnoumber ==0
decaytime =1;
conductancemaximum =0;
else
decaytime = decaytimes1(6, eventnoumber);
conductancemaximum = conductancemaxima1(6, eventnoumber);
end

== matlab function pattern_separation/granule cell 6/MATLAB Function2 ==
  data: eventnoumber input; decaytime output; decaytimes2 input; conductancemaxima2 input; conductancemaximum output
function [decaytime, conductancemaximum] = fcn(eventnoumber, decaytimes2, conductancemaxima2)
if eventnoumber ==0
decaytime =1;
conductancemaximum =0;
else
decaytime = decaytimes2(6, eventnoumber);
conductancemaximum = conductancemaxima2(6, eventnoumber);
end

== matlab function pattern_separation/granule cell 6/single exp EPSCs generator (recurrent synapse)/MATLAB Function ==
  data: inp input; exponential output
function exponential = fcn(inp)

exponential = exp(-inp);

== matlab function pattern_separation/granule cell 6/single exp IPSCs generator (ihibitory synapse)/MATLAB Function ==
  data: inp input; exponential output
function exponential = fcn(inp)

exponential = exp(-inp);

== matlab function pattern_separation/granule cell 7/MATLAB Function1 ==
  data: eventnoumber input; decaytime output; decaytimes1 input; conductancemaxima1 input; conductancemaximum output
function [decaytime, conductancemaximum] = fcn(eventnoumber, decaytimes1, conductancemaxima1)
if eventnoumber ==0
decaytime =1;
conductancemaximum =0;
else
decaytime = decaytimes1(7, eventnoumber);
conductancemaximum = conductancemaxima1(7, eventnoumber);
end

== matlab function pattern_separation/granule cell 7/MATLAB Function2 ==
  data: eventnoumber input; decaytime output; decaytimes2 input; conductancemaxima2 input; conductancemaximum output
function [decaytime, conductancemaximum] = fcn(eventnoumber, decaytimes2, conductancemaxima2)
if eventnoumber ==0
decaytime =1;
conductancemaximum =0;
else
decaytime = decaytimes2(7, eventnoumber);
conductancemaximum = conductancemaxima2(7, eventnoumber);
end

== matlab function pattern_separation/granule cell 7/granule cell/reset function ==
  data: v input; c input; d input; u input; v1 output; u1 output; r output

function [v1,u1,r] = fcn(v,c,d,u)

if v >= 30
v1= c;
u1 = u+d;
r=1;
else
v1=v;
u1=u;
r=0;  
end

== matlab function pattern_separation/granule cell 7/single exp EPSCs generator (recurrent synapse)/MATLAB Function ==
  data: inp input; exponential output
function exponential = fcn(inp)

exponential = exp(-inp);

== matlab function pattern_separation/granule cell 7/single exp IPSCs generator (ihibitory synapse)/MATLAB Function ==
  data: inp input; exponential output
function exponential = fcn(inp)

exponential = exp(-inp);

== matlab function pattern_separation/granule cell 8/GC neuron/reset function ==
  data: v input; c input; d input; u input; v1 output; u1 output; r output

function [v1,u1,r] = fcn(v,c,d,u)

if v >= 30
v1= c;
u1 = u+d;
r=1;
else
v1=v;
u1=u;
r=0;  
end

== matlab function pattern_separation/granule cell 8/MATLAB Function1 ==
  data: eventnoumber input; decaytime output; decaytimes1 input; conductancemaxima1 input; conductancemaximum output
function [decaytime, conductancemaximum] = fcn(eventnoumber, decaytimes1, conductancemaxima1)
if eventnoumber ==0
decaytime =1;
conductancemaximum =0;
else
decaytime = decaytimes1(8, eventnoumber);
conductancemaximum = conductancemaxima1(8, eventnoumber);
end

== matlab function pattern_separation/granule cell 8/MATLAB Function2 ==
  data: eventnoumber input; decaytime output; decaytimes2 input; conductancemaxima2 input; conductancemaximum output
function [decaytime, conductancemaximum] = fcn(eventnoumber, decaytimes2, conductancemaxima2)
if eventnoumber ==0
decaytime =1;
conductancemaximum =0;
else
decaytime = decaytimes2(8, eventnoumber);
conductancemaximum = conductancemaxima2(8, eventnoumber);
end

== matlab function pattern_separation/granule cell 8/single exp EPSCs generator (recurrent synapse)/MATLAB Function ==
  data: inp input; exponential output
function exponential = fcn(inp)

exponential = exp(-inp);

== matlab function pattern_separation/granule cell 8/single exp IPSCs generator (ihibitory synapse)/MATLAB Function ==
  data: inp input; exponential output
function exponential = fcn(inp)

exponential = exp(-inp);

== matlab function pattern_separation/granule cell 10/GC neuron/reset function ==
  data: v input; c input; d input; u input; v1 output; u1 output; r output

function [v1,u1,r] = fcn(v,c,d,u)

if v >= 30
v1= c;
u1 = u+d;
r=1;
else
v1=v;
u1=u;
r=0;  
end

== matlab function pattern_separation/granule cell 10/MATLAB Function1 ==
  data: eventnoumber input; decaytime output; decaytimes1 input; conductancemaxima1 input; conductancemaximum output
function [decaytime, conductancemaximum] = fcn(eventnoumber, decaytimes1, conductancemaxima1)
if eventnoumber ==0
decaytime =1;
conductancemaximum =0;
else
decaytime = decaytimes1(10, eventnoumber);
conductancemaximum = conductancemaxima1(10, eventnoumber);
end

== matlab function pattern_separation/granule cell 10/MATLAB Function2 ==
  data: eventnoumber input; decaytime output; decaytimes2 input; conductancemaxima2 input; conductancemaximum output
function [decaytime, conductancemaximum] = fcn(eventnoumber, decaytimes2, conductancemaxima2)
if eventnoumber ==0
decaytime =1;
conductancemaximum =0;
else
decaytime = decaytimes2(1, eventnoumber);
conductancemaximum = conductancemaxima2(1, eventnoumber);
end

== matlab function pattern_separation/granule cell 10/single exp EPSCs generator (recurrent synapse)/MATLAB Function ==
  data: inp input; exponential output
function exponential = fcn(inp)

exponential = exp(-inp);

== matlab function pattern_separation/granule cell 10/single exp IPSCs generator (ihibitory synapse)/MATLAB Function ==
  data: inp input; exponential output
function exponential = fcn(inp)

exponential = exp(-inp);

== matlab function pattern_separation/granule cell 11/MATLAB Function1 ==
  data: eventnoumber input; decaytime output; decaytimes1 input; conductancemaxima1 input; conductancemaximum output
function [decaytime, conductancemaximum] = fcn(eventnoumber, decaytimes1, conductancemaxima1)
if eventnoumber ==0
decaytime =1;
conductancemaximum =0;
else
decaytime = decaytimes1(11, eventnoumber);
conductancemaximum = conductancemaxima1(11, eventnoumber);
end

== matlab function pattern_separation/granule cell 11/MATLAB Function2 ==
  data: eventnoumber input; decaytime output; decaytimes2 input; conductancemaxima2 input; conductancemaximum output
function [decaytime, conductancemaximum] = fcn(eventnoumber, decaytimes2, conductancemaxima2)
if eventnoumber ==0
decaytime =1;
conductancemaximum =0;
else
decaytime = decaytimes2(11, eventnoumber);
conductancemaximum = conductancemaxima2(11, eventnoumber);
end

== matlab function pattern_separation/granule cell 11/granule cell/reset function ==
  data: v input; c input; d input; u input; v1 output; u1 output; r output

function [v1,u1,r] = fcn(v,c,d,u)

if v >= 30
v1= c;
u1 = u+d;
r=1;
else
v1=v;
u1=u;
r=0;  
end

== matlab function pattern_separation/granule cell 11/single exp EPSCs generator (recurrent synapse)/MATLAB Function ==
  data: inp input; exponential output
function exponential = fcn(inp)

exponential = exp(-inp);

== matlab function pattern_separation/granule cell 11/single exp IPSCs generator (ihibitory synapse)/MATLAB Function ==
  data: inp input; exponential output
function exponential = fcn(inp)

exponential = exp(-inp);

== matlab function pattern_separation/granule cell 12/GC neuron/reset function ==
  data: v input; c input; d input; u input; v1 output; u1 output; r output

function [v1,u1,r] = fcn(v,c,d,u)

if v >= 30
v1= c;
u1 = u+d;
r=1;
else
v1=v;
u1=u;
r=0;  
end

== matlab function pattern_separation/granule cell 12/MATLAB Function1 ==
  data: eventnoumber input; decaytime output; decaytimes1 input; conductancemaxima1 input; conductancemaximum output
function [decaytime, conductancemaximum] = fcn(eventnoumber, decaytimes1, conductancemaxima1)
if eventnoumber ==0
decaytime =1;
conductancemaximum =0;
else
decaytime = decaytimes1(12, eventnoumber);
conductancemaximum = conductancemaxima1(12, eventnoumber);
end

== matlab function pattern_separation/granule cell 12/MATLAB Function2 ==
  data: eventnoumber input; decaytime output; decaytimes2 input; conductancemaxima2 input; conductancemaximum output
function [decaytime, conductancemaximum] = fcn(eventnoumber, decaytimes2, conductancemaxima2)
if eventnoumber ==0
decaytime =1;
conductancemaximum =0;
else
decaytime = decaytimes2(12, eventnoumber);
conductancemaximum = conductancemaxima2(12, eventnoumber);
end

== matlab function pattern_separation/granule cell 12/single exp EPSCs generator (recurrent synapse)/MATLAB Function ==
  data: inp input; exponential output
function exponential = fcn(inp)

exponential = exp(-inp);

== matlab function pattern_separation/granule cell 12/single exp IPSCs generator (ihibitory synapse)/MATLAB Function ==
  data: inp input; exponential output
function exponential = fcn(inp)

exponential = exp(-inp);
